simulink model "Block_Commutation"  (R2013b)
settings: Solver=ode45  StartTime=0.0  StopTime=10  RelTol=1e-3
libraries: nesl_utility x10, fl_lib x8, pe_lib x7, simulink x6, elec_lib x3, powerlib_meascontrol x1
settings Model: Creator=Eduardo  LastModifiedBy=Eduardo

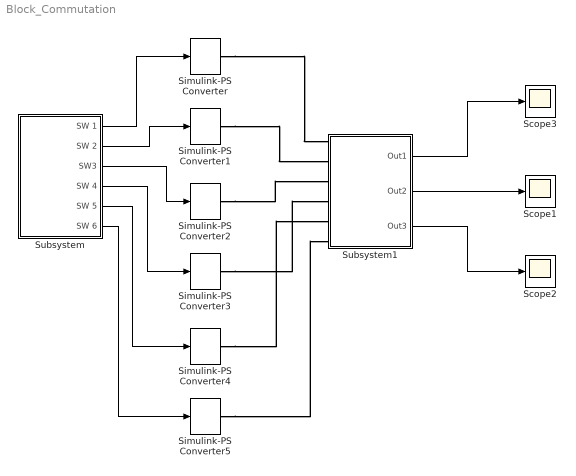
== system Block_Commutation ==
  Scope1 : Scope
      settings: TimeRange=1  YMin=0  YMax=1  SaveName=ScopeData4
  Scope2 : Scope
      settings: TimeRange=1.5  YMin=0  YMax=6  SaveName=ScopeData5
  Scope3 : Scope
      settings: TimeRange=1  YMin=0  YMax=1
  Simulink-PS Converter{,1..5} (6 alike) : nesl_utility/Simulink-PS Converter  PhysicalDomain=network_engine_domain  SubClassName=ps_input  LeftPortType=input  RightPortType=output  PseudoPeriodic=off  Frequencies=[]  NoiseDistribution=none  NoiseParameters=[]  Unit=1  AffineConversion=off  InputFiltering=off  SimscapeFilterOrder=1  InputFilterTimeConstant=0.001  UdotUserProvided=1
  Subsystem : Subsystem
  Subsystem1 : Subsystem
  wires:
  Subsystem/1(SW 1) -> Simulink-PS Converter/1
  Subsystem/2(SW 2) -> Simulink-PS Converter1/1
  Subsystem/3("SW3 ") -> Simulink-PS Converter2/1
  Subsystem/4(SW 4) -> Simulink-PS Converter3/1
  Subsystem/5(SW 5) -> Simulink-PS Converter4/1
  Subsystem/6(SW 6) -> Simulink-PS Converter5/1
  Subsystem1/2(Out2) -> Scope1/1
  Subsystem1/3(Out3) -> Scope2/1
  Subsystem1/1(Out1) -> Scope3/1
  connections:
  Simulink-PS Converter2/RConn1 -- Subsystem1/LConn3
  Simulink-PS Converter1/RConn1 -- Subsystem1/LConn2
  Simulink-PS Converter3/RConn1 -- Subsystem1/LConn4
  Simulink-PS Converter/RConn1 -- Subsystem1/LConn1
  Simulink-PS Converter4/RConn1 -- Subsystem1/LConn5
  Simulink-PS Converter5/RConn1 -- Subsystem1/LConn6

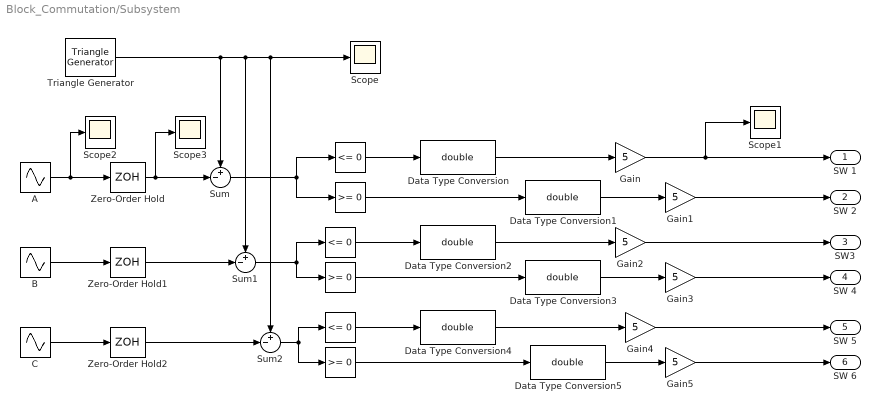
== system Block_Commutation/Subsystem ==
  " " : simulink/Logic and Bit Operations/Compare To Zero  relop=<=  OutDataTypeStr=boolean
  "  " : simulink/Logic and Bit Operations/Compare To Zero  relop=<=  OutDataTypeStr=boolean
  "    " : simulink/Logic and Bit Operations/Compare To Zero  relop=<=  OutDataTypeStr=boolean
  "      " : simulink/Logic and Bit Operations/Compare To Zero  relop=>=  OutDataTypeStr=boolean
  "                      " : simulink/Logic and Bit Operations/Compare To Zero  relop=>=  OutDataTypeStr=boolean
  "                       " : simulink/Logic and Bit Operations/Compare To Zero  relop=>=  OutDataTypeStr=boolean
  A : Sin  Frequency=10  SampleTime=0
  B : Sin  Frequency=10  Phase=3*pi/4  SampleTime=0
  C : Sin  Frequency=10  Phase=6*pi/4  SampleTime=0
  Data Type Conversion{,1..5} (6 alike) : DataTypeConversion  OutDataTypeStr=double  LockScale=on
  Gain{,1..5} (6 alike) : Gain  Gain=5
  Scope{,1..3} (4 alike) : Scope
      Scope1 settings: TimeRange=1  YMin=0  YMax=1  SaveName=ScopeData6
      Scope2 settings: TimeRange=1  YMin=0  YMax=1  SaveName=ScopeData2
      Scope3 settings: TimeRange=1  YMin=0  YMax=1  SaveName=ScopeData3
  Sum : Sum  Inputs=+-|
  Sum1 : Sum  Inputs=+-|
  Sum2 : Sum  Inputs=+-|
  Triangle Generator : powerlib_meascontrol/Pulse & Signal Generators/Triangle Generator  Freq=100  Phase=90  Ts=0
  Zero-Order Hold : ZeroOrderHold  SampleTime=10^-3
  Zero-Order Hold1 : ZeroOrderHold  SampleTime=10^-3
  Zero-Order Hold2 : ZeroOrderHold  SampleTime=10^-3
  SW 1 : Outport
  SW 2 : Outport  Port=2
  "SW3 " : Outport  Port=3
  SW 4 : Outport  Port=4
  SW 5 : Outport  Port=5
  SW 6 : Outport  Port=6
  wires:
  Sum/1 -> "      "/1, " "/1
  B/1 -> Zero-Order Hold1/1
  C/1 -> Zero-Order Hold2/1
  Sum1/1 -> "                       "/1, "  "/1
  Triangle Generator/1 -> Scope/1, Sum2/1, Sum1/1, Sum/1
  "                      "/1 -> Data Type Conversion5/1
  "    "/1 -> Data Type Conversion4/1
  "  "/1 -> Data Type Conversion2/1
  "                       "/1 -> Data Type Conversion3/1
  "      "/1 -> Data Type Conversion1/1
  " "/1 -> Data Type Conversion/1
  Sum2/1 -> "    "/1, "                      "/1
  Zero-Order Hold/1 -> Scope3/1, Sum/2
  A/1 -> Scope2/1, Zero-Order Hold/1
  Zero-Order Hold1/1 -> Sum1/2
  Zero-Order Hold2/1 -> Sum2/2
  Data Type Conversion/1 -> Gain/1
  Data Type Conversion1/1 -> Gain1/1
  Data Type Conversion2/1 -> Gain2/1
  Data Type Conversion3/1 -> Gain3/1
  Data Type Conversion4/1 -> Gain4/1
  Data Type Conversion5/1 -> Gain5/1
  Gain/1 -> Scope1/1, SW 1/1
  Gain1/1 -> SW 2/1
  Gain2/1 -> "SW3 "/1
  Gain3/1 -> SW 4/1
  Gain4/1 -> SW 5/1
  Gain5/1 -> SW 6/1

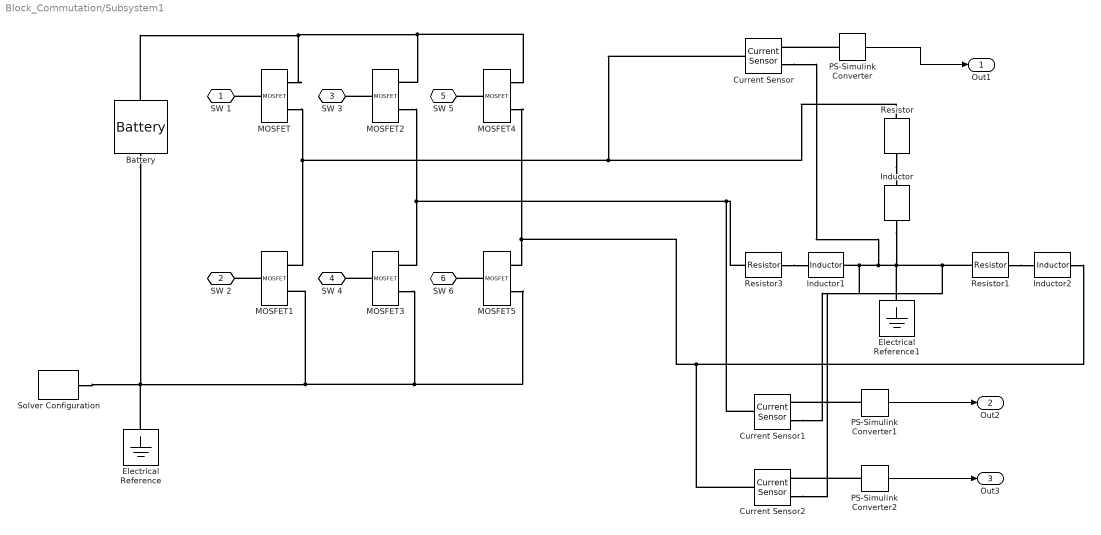
== system Block_Commutation/Subsystem1 ==
  Battery : pe_lib/Sources/Battery  Vnom=12 V  AH=50 hr*A  AH0=50 hr*A  V1=11.5 V  AH1=25 hr*A  R1=2 Ohm  R2=inf Ohm  alpha=1  beta=1  G2=0 S  i_Log=off  charge_Log=off  LocalVarNames=|i|charge  LocalVarDescs=|i|Charge state  LocalVarLogging=[0 0]
  Current Sensor : fl_lib/Electrical/Electrical Sensors/Current Sensor  i1_Log=off  v1_Log=off  LocalVarNames=|i1|v1  LocalVarDescs=|i1|v1  LocalVarLogging=[0 0]
  Current Sensor1 : fl_lib/Electrical/Electrical Sensors/Current Sensor  i1_Log=off  v1_Log=off  LocalVarNames=|i1|v1  LocalVarDescs=|i1|v1  LocalVarLogging=[0 0]
  Current Sensor2 : fl_lib/Electrical/Electrical Sensors/Current Sensor  i1_Log=off  v1_Log=off  LocalVarNames=|i1|v1  LocalVarDescs=|i1|v1  LocalVarLogging=[0 0]
  Electrical Reference : fl_lib/Electrical/Electrical Elements/Electrical Reference  i_Log=off  LocalVarNames=|i  LocalVarDescs=|i  LocalVarLogging=0
  Electrical Reference1 : fl_lib/Electrical/Electrical Elements/Electrical Reference  i_Log=off  LocalVarNames=|i  LocalVarDescs=|i  LocalVarLogging=0
  Inductor : fl_lib/Electrical/Electrical Elements/Inductor  l=0.322 mH  i0=0 A  r=0 Ohm  g=1e-9 1/Ohm  i_Log=off  v_Log=off  i_L_Log=off  LocalVarNames=|i|v|i_L  LocalVarDescs=|i|v|Internal variable for current through inductor term  LocalVarLogging=[0 0 0]
  Inductor1 : fl_lib/Electrical/Electrical Elements/Inductor  l=0.322 mH  i0=0 A  r=0 Ohm  g=1e-9 1/Ohm  i_Log=off  v_Log=off  i_L_Log=off  LocalVarNames=|i|v|i_L  LocalVarDescs=|i|v|Internal variable for current through inductor term  LocalVarLogging=[0 0 0]
  Inductor2 : fl_lib/Electrical/Electrical Elements/Inductor  l=0.322 mH  i0=0 A  r=0 Ohm  g=1e-9 1/Ohm  i_Log=off  v_Log=off  i_L_Log=off  LocalVarNames=|i|v|i_L  LocalVarDescs=|i|v|Internal variable for current through inductor term  LocalVarLogging=[0 0 0]
  MOSFET{,1..5} (6 alike) : pe_lib/Semiconductors/Fundamental Components/MOSFET  Rds=0.01 Ohm  Goff=1e-6 1/Ohm  Vth=2 V  diode_param=2  diode_Vf=0.8 V  diode_Ron=0.001 Ohm  diode_Goff=1e-5 1/Ohm  diode_C=5e-8 F  diode_iRM=-235 A  diode_iF=300 A  diode_idot=-50 A/us  diode_trr_param=1  diode_trr_factor=3  diode_trr=15 us  diode_Qrr=1.5e+3 s*uA  LocalVarLogging=[]
  PS-Simulink Converter : nesl_utility/PS-Simulink Converter  PhysicalDomain=network_engine_domain  SubClassName=ps_output  LeftPortType=input  RightPortType=output  PseudoPeriodic=off  Frequencies=[]  Unit=1  AffineConversion=off
  PS-Simulink Converter1 : nesl_utility/PS-Simulink Converter  PhysicalDomain=network_engine_domain  SubClassName=ps_output  LeftPortType=input  RightPortType=output  PseudoPeriodic=off  Frequencies=[]  Unit=1  AffineConversion=off
  PS-Simulink Converter2 : nesl_utility/PS-Simulink Converter  PhysicalDomain=network_engine_domain  SubClassName=ps_output  LeftPortType=input  RightPortType=output  PseudoPeriodic=off  Frequencies=[]  Unit=1  AffineConversion=off
  Resistor : elec_lib/Passive Devices/Resistor  R=0.463 Ohm  noise_mode=0  Tdevice=25 C  sample_time=0.001 s  repeatability=1  auto_seed=2517246261  user_seed=0  LocalVarLogging=[]
  Resistor1 : elec_lib/Passive Devices/Resistor  R=0.463 Ohm  noise_mode=0  Tdevice=25 C  sample_time=0.001 s  repeatability=1  auto_seed=3215666574  user_seed=0  LocalVarLogging=[]
  Resistor3 : elec_lib/Passive Devices/Resistor  R=0.463 Ohm  noise_mode=0  Tdevice=25 C  sample_time=0.001 s  repeatability=1  auto_seed=1747857717  user_seed=0  LocalVarLogging=[]
  Solver Configuration : nesl_utility/Solver Configuration  PhysicalDomain=network_engine_domain  SubClassName=solver  LeftPortType=input  RightPortType=generic  Accelerate=off  Tones=[]  Harmonics=[]  SimulateNoise=off  Profile=off  UseLocalSampling=off  EnableSwitchedLinearOptims=on  FrequencyDomain=off  UseCCode=off  RelTol=0.001  AbsTol=1e-06  MinStep=1e-09  ToWorkspace=off  DoDC=off  ResidualTolerance=1e-09  UseLocalSolver=off  LocalSolverChoice=NE_BACKWARD_EULER_ADVANCER  LocalSolverSampleTime=0.001  DoFixedCost=off  MaxNonlinIter=3  MaxModeIter=2  LinearAlgebra=Sparse  DelaysMemoryBudget=1024
  "SW 1 " : PMIOPort  Port=1  Side=Left
  SW 2 : PMIOPort  Port=2  Side=Left
  SW 3 : PMIOPort  Port=3  Side=Left
  SW 4 : PMIOPort  Port=4  Side=Left
  SW 5 : PMIOPort  Port=5  Side=Left
  SW 6 : PMIOPort  Port=6  Side=Left
  Out1 : Outport
  Out2 : Outport  Port=2
  Out3 : Outport  Port=3
  wires:
  PS-Simulink Converter/1 -> Out1/1
  PS-Simulink Converter1/1 -> Out2/1
  PS-Simulink Converter2/1 -> Out3/1
  connections:
  MOSFET/RConn1 -- Battery/LConn1 -- MOSFET4/RConn1 -- MOSFET2/RConn1
  MOSFET/RConn2 -- Resistor/LConn1 -- Current Sensor/LConn1 -- MOSFET1/RConn1
  MOSFET5/RConn2 -- MOSFET3/RConn2 -- Electrical Reference/LConn1 -- Solver Configuration/RConn1 -- Battery/RConn1 -- MOSFET1/RConn2
  MOSFET/LConn1 -- "SW 1 "/RConn1
  MOSFET4/LConn1 -- SW 5/RConn1
  MOSFET5/LConn1 -- SW 6/RConn1
  MOSFET3/LConn1 -- SW 4/RConn1
  MOSFET1/LConn1 -- SW 2/RConn1
  MOSFET2/LConn1 -- SW 3/RConn1
  MOSFET4/RConn2 -- Current Sensor2/LConn1 -- Inductor2/RConn1 -- MOSFET5/RConn1
  MOSFET2/RConn2 -- Current Sensor1/LConn1 -- Resistor3/LConn1 -- MOSFET3/RConn1
  Resistor/RConn1 -- Inductor/LConn1
  Resistor3/RConn1 -- Inductor1/LConn1
  Resistor1/RConn1 -- Inductor2/LConn1
  Inductor/RConn1 -- Current Sensor2/RConn2 -- Resistor1/LConn1 -- Electrical Reference1/LConn1 -- Current Sensor/RConn2 -- Current Sensor1/RConn2 -- Inductor1/RConn1
  PS-Simulink Converter/LConn1 -- Current Sensor/RConn1
  PS-Simulink Converter1/LConn1 -- Current Sensor1/RConn1
  PS-Simulink Converter2/LConn1 -- Current Sensor2/RConn1
